simulink model "PS1_simulink"  (R2024b)
settings: Solver=FixedStepAuto  StartTime=0  StopTime=s/12  FixedStep=dt  RelTol=1e-3
InitFcn:
  | s = 86400;
  | dt = 1;

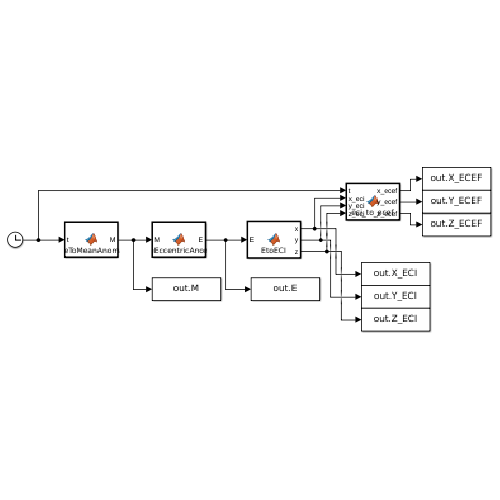
[thumbnail: Simulink's stored preview of the top-level diagram]
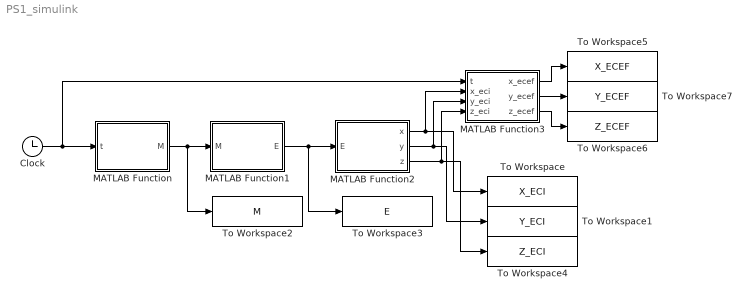
== system PS1_simulink ==
  Clock : Clock
      settings: Decimation=100
  MATLAB Function : MATLAB Function  TreatAsAtomicUnit=on
  MATLAB Function1 : MATLAB Function  TreatAsAtomicUnit=on
  MATLAB Function2 : MATLAB Function  TreatAsAtomicUnit=on
  MATLAB Function3 : MATLAB Function  TreatAsAtomicUnit=on
  To Workspace : ToWorkspace  VariableName=X_ECI  SaveFormat=Timeseries  SampleTime=-1
  To Workspace1 : ToWorkspace  VariableName=Y_ECI  SaveFormat=Timeseries  SampleTime=-1
  To Workspace2 : ToWorkspace  VariableName=M  SaveFormat=Timeseries  SampleTime=-1
  To Workspace3 : ToWorkspace  VariableName=E  SaveFormat=Timeseries  SampleTime=-1
  To Workspace4 : ToWorkspace  VariableName=Z_ECI  SaveFormat=Timeseries  SampleTime=-1
  To Workspace5 : ToWorkspace  VariableName=X_ECEF  SaveFormat=Timeseries  SampleTime=-1
  To Workspace6 : ToWorkspace  VariableName=Z_ECEF  SaveFormat=Timeseries  SampleTime=-1
  To Workspace7 : ToWorkspace  VariableName=Y_ECEF  SaveFormat=Timeseries  SampleTime=-1
  wires:
  Clock/1 -> MATLAB Function3/1(t), MATLAB Function/1(t)
  MATLAB Function/1(M) -> To Workspace2/1, MATLAB Function1/1(M)
  MATLAB Function1/1(E) -> To Workspace3/1, MATLAB Function2/1(E)
  MATLAB Function2/1(x) -> MATLAB Function3/2(x_eci), To Workspace/1
  MATLAB Function2/2(y) -> MATLAB Function3/3(y_eci), To Workspace1/1
  MATLAB Function2/3(z) -> MATLAB Function3/4(z_eci), To Workspace4/1
  MATLAB Function3/1(x_ecef) -> To Workspace5/1
  MATLAB Function3/2(y_ecef) -> To Workspace7/1
  MATLAB Function3/3(z_ecef) -> To Workspace6/1

== matlab function PS1_simulink/MATLAB Function1 ==
  data: M input; E output
function E = solveEccentricAnomaly(M)
    
    e = 0.0001971;
    epsilon = 1*10^(-8);
    E = pi;

    while true
        f  = E - e * sin(E) - M;
        fp = 1 - e * cos(E);
        
        E_new = E - f / fp;
        
        if abs(E_new - E) < epsilon
            break;
        end
        
        E = E_new;
    end
end

== matlab function PS1_simulink/MATLAB Function ==
  data: t input; M output
function M  = timeToMeanAnomaly(t)
    mu = 3.986*10^5;
    a = 7155.81;
    M0 = deg2rad(267.074);
    n = sqrt(mu/a^3);
    M = wrapTo2Pi(M0 + n*t);
end

== matlab function PS1_simulink/MATLAB Function2 ==
  data: x output; E input; y output; z output
function [x,y,z] = EtoECI(E)

a = 7155.81;
e = 0.0001971;
i = deg2rad(86.403);
Omega = deg2rad(230.875);
omega = deg2rad(93.069);

r_p = [a*(cos(E)-e), a*sqrt(1-e^2)*sin(E), 0.0];

R11 = cos(Omega) * cos(omega) - sin(Omega) * sin(omega) * cos(i);
R12 = -cos(Omega) * sin(omega) - sin(Omega) * cos(omega) * cos(i);
R13 = sin(Omega) * sin(i);

R21 = sin(Omega) * cos(omega) + cos(Omega) * sin(omega) * cos(i);
R22 = -sin(Omega) * sin(omega) + cos(Omega) * cos(omega) * cos(i);
R23 = -cos(Omega) * sin(i);

R31 = sin(omega) * sin(i);
R32 = cos(omega) * sin(i);
R33 = cos(i);

R = [R11, R12, R13;
     R21, R22, R23;
     R31, R32, R33];

r_ECI = R * r_p';
x = r_ECI(1);
y = r_ECI(2);
z = r_ECI(3);
end

== matlab function PS1_simulink/MATLAB Function3 ==
  data: t input; x_ecef output; x_eci input; y_ecef output; z_ecef output; y_eci input; z_eci input
function [x_ecef, y_ecef, z_ecef] = eci_to_ecef(t, x_eci, y_eci, z_eci)

    omega_earth = 7.2921159e-5;
    theta_0 = 0.2603;
    dUT1 = -0.01423;
    theta = theta_0 + omega_earth*(t+dUT1);

    R = [cos(theta), sin(theta), 0;
        -sin(theta), cos(theta), 0;
        0, 0, 1];

    r_eci = [x_eci; y_eci; z_eci];
    r_ecef = R * r_eci;

    x_ecef = r_ecef(1);
    y_ecef = r_ecef(2);
    z_ecef = r_ecef(3);
end
